simulink model "DisertatieVanca"  (R2022b)
settings: Solver=FixedStepAuto  StartTime=0.0  StopTime=10.0  RelTol=1e-3
values from neighbouring files (symbols this model uses):
  Ts = T_pwm    (= 0.001)    [RLagent.m]
  Ts_agent = Ts    (= 0.001)    [RLagent.m]
  Ts_speed = 10*Ts    (= 0.01)    [RLagent.m]
undefined symbols (not defined in the file or in its folder): DiscIntNeverNeededParam, Ion, Lithium
libraries: spsSeriesRLCBranchLib x10, spsDiodeLib x7, spsIGBTLib x6, mcbcontrolslib x3, simulink x3, spsVoltageMeasurementLib x3, spsThreePhaseVIMeasurementLib x3, spsCurrentMeasurementLib x2, spsBatteryLib x1, BatteryEstimators x1, spsIGBTDiodeLib x1, slpidlib x1
(part 1 of 2)
settings Model: Creator=uiv66426  LastModifiedBy=uiv66426
settings DebuggingCC: ParameterOverflowMsg=none  ParameterUnderflowMsg=error  ParameterPrecisionLossMsg=none
settings HardwareCC: TargetBitPerPointer=64  TargetBitPerSizeT=64  TargetBitPerPtrDiffT=64  TargetLongLongMode=on  TargetIntDivRoundTo=Zero  TargetEndianess=LittleEndian  TargetWordSize=64  TargetHWDeviceType=MATLAB Host  ProdEqTarget=off
settings RTWCC: Description=Rapid Simulation Target  SystemTargetFile=rsim.tlc  TemplateMakefile=rsim_default_tmf
settings RSimTargetCC: TargetLangStandard=C99 (ISO)  OptimizeReductions=off

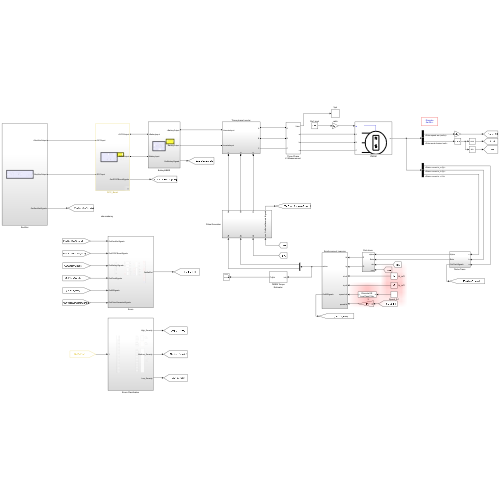
[thumbnail: Simulink's stored preview of the top-level diagram]
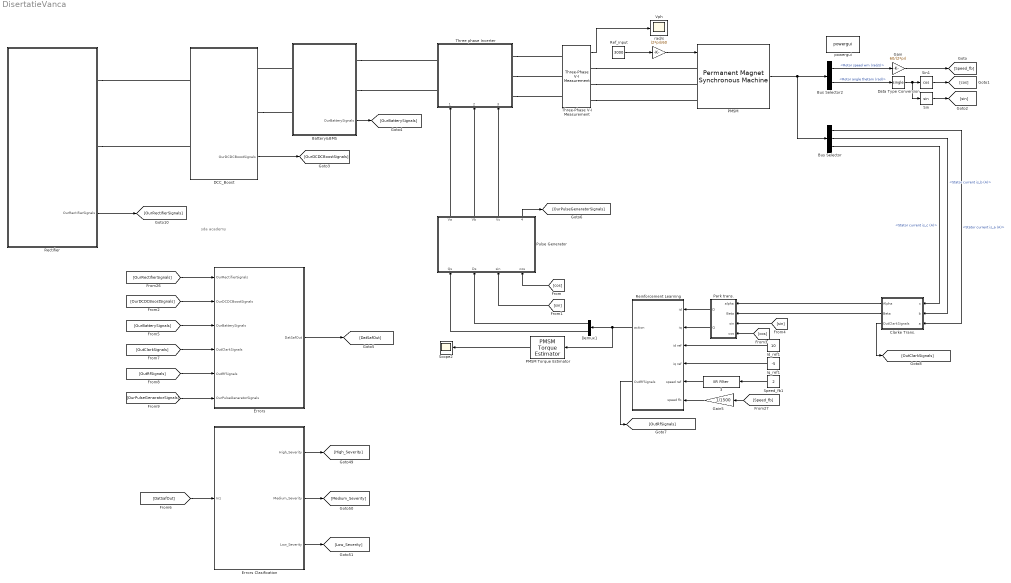
== system DisertatieVanca ==
  note: sda academy
  "   3" : mcbcontrolslib/IIR Filter  VariantControl=Low Pass Filter  VariantSelect=Low-pass  Filter_constant=0.01*(Ts_speed/Ts)  advancedSettings=off  Ts=50e-6  cutOff_freq=1
  Battery&BMS : Subsystem
      settings: PortSchema="{\"entries\":[{\"content\":{\"sides\":[{\"content\":{\"connectorIds\":[\"LConn1\",\"LConn2\"]},\"type\":\"ConnectorPlacement.EquallySpacedRectSide\",\"uuid\":\"cbc0bb53-0b94-40dd-8246-9b05db34f507\"},{\"content\":{\"connectorIds\":[\"RConn1\",\"RConn2\",\"Out1\"],\"side\":\"RIGHT\"},\"type\":\"ConnectorPlacement.EquallySpacedRectSide\",\"uuid\":\"2d021873-454e-497b-a321-1833202da2b2\"},{\"content\":{\"connectorIds\":[],\"side\":\"TOP\"},\"type\":\"ConnectorPlacement.EquallySpacedRectSide\",\"uuid\":\"d1b949f0-43da-4a40-bdda-1f67f09c131a\"}]},\"type\":\"ConnectorPlacement.EquallySpacedConnector\",\"uuid\":\"de95084d-4868-446f-8974-e187dacb7426\"}],\"packageUris\":[\"http://schema.mathworks.com/mf0/Connector/R2020b\"],\"version\":\"1.0\"}"
  Bus Selector : BusSelector  OutputSignals=Stator current is_a (A),Stator current is_b (A),Stator current is_c (A)
  Bus Selector2 : BusSelector  OutputSignals=Rotor speed wm (rad/s),Rotor angle thetam (rad)
  Clarke Trans. : Subsystem
  DCC_Boost : Subsystem
      settings: PortSchema="{\"entries\":[{\"content\":{\"sides\":[{\"content\":{\"connectorIds\":[\"LConn1\",\"LConn2\"]},\"type\":\"ConnectorPlacement.EquallySpacedRectSide\",\"uuid\":\"cbc0bb53-0b94-40dd-8246-9b05db34f507\"},{\"content\":{\"connectorIds\":[\"RConn1\",\"RConn2\",\"Out1\"],\"side\":\"RIGHT\"},\"type\":\"ConnectorPlacement.EquallySpacedRectSide\",\"uuid\":\"2d021873-454e-497b-a321-1833202da2b2\"},{\"content\":{\"connectorIds\":[],\"side\":\"TOP\"},\"type\":\"ConnectorPlacement.EquallySpacedRectSide\",\"uuid\":\"d1b949f0-43da-4a40-bdda-1f67f09c131a\"}]},\"type\":\"ConnectorPlacement.EquallySpacedConnector\",\"uuid\":\"de95084d-4868-446f-8974-e187dacb7426\"}],\"packageUris\":[\"http://schema.mathworks.com/mf0/Connector/R2020b\"],\"version\":\"1.0\"}"
  Data Type Conversion : DataTypeConversion  OutDataTypeStr=single  SaturateOnIntegerOverflow=off  RndMeth=Floor
  Demux1 : Demux  Outputs=2
  Errors : Subsystem
  Errors Clasification : Subsystem
  Gain : Gain  Gain=60/(2*pi)  OutDataTypeStr=double
  Gain5 : Gain  Gain=1/1500
  Id_ref1 : Constant  Value=10  OutDataTypeStr=double  SampleTime=Ts_speed
  Iq_ref1 : Constant  Value=-5  OutDataTypeStr=double  SampleTime=Ts_speed
  PMSM : spsPermanentMagnetSynchronousMachineLib/Permanent Magnet Synchronous Machine  NbPhases=3  FluxDistribution=Sinusoidal  RotorType=Salient-pole  MechanicalLoad=Speed w  PresetModel=No  ShowDetailedParameters=on  MeasurementBus=off  Resistance=18.7  Inductance=8.5e-3  dqInductances=[0.02547 0.02816]  La=0.000395  MachineConstant=Flux linkage established by magnets (V.s)  Flux=0.1716  VoltageCst=62.2496  TorqueCst=0.5148  Flat=120  Mechanical=[2.26e-05 1.349e-05 2 0]  PolePairs=2  InitialConditions=[0,0, 0,0]  InitialConditions5ph=[0 0 0 0 0 0]  RefAngle=Aligned with phase A axis (original Park)  IterativeDiscreteModel=Trapezoidal non iterative  TsBlock=-1  TsPowergui=0
  PMSM Torque Estimator : eePmsmTorqueEstimator/PMSM Torque Estimator  ParamType=Constant parameters  p=8  idVect=[-200, 200]  iqVect=[-200, 200]  LdMatrix=0.0002 * ones(2, 2)  LqMatrix=0.0002 * ones(2, 2)  psimMatrix=0.04 * ones(2, 2)  Ld=0.0002  Lq=0.0002  psim=0.04  Ts=-1
  Park trans. : Subsystem
  Pulse Generator : Subsystem
  Rectifier : Subsystem
      settings: PortSchema="{\"entries\":[{\"content\":{\"sides\":[{\"content\":{\"connectorIds\":[]},\"type\":\"ConnectorPlacement.EquallySpacedRectSide\",\"uuid\":\"7d3ba707-0ee8-4d26-a752-be0b8f38d830\"},{\"content\":{\"connectorIds\":[\"RConn1\",\"RConn2\",\"Out1\"],\"side\":\"RIGHT\"},\"type\":\"ConnectorPlacement.EquallySpacedRectSide\",\"uuid\":\"4da73b4e-8794-485b-9d0a-8f3b9b630819\"},{\"content\":{\"connectorIds\":[],\"side\":\"TOP\"},\"type\":\"ConnectorPlacement.EquallySpacedRectSide\",\"uuid\":\"189264b5-1a07-455a-ade0-b52dce53e5ab\"}]},\"type\":\"ConnectorPlacement.EquallySpacedConnector\",\"uuid\":\"df5a9191-3afb-48d4-8cb4-bd3682c9bea9\"}],\"packageUris\":[\"http://schema.mathworks.com/mf0/Connector/R2020b\"],\"version\":\"1.0\"}"
  Ref_input : Constant  Value=3000  SampleTime=0.0005
  Reinforcement Learning : Subsystem
  Scope2 : Scope
  Sin : Trigonometry  NumberOfDataPoints=double
  Sin1 : Trigonometry  Operator=cos
  Speed_fb1 : Constant  Value=2  SampleTime=Ts_speed
  Three phase Inverter : Subsystem
      settings: PortSchema="{\"entries\":[{\"content\":{\"sides\":[{\"content\":{\"connectorIds\":[\"LConn1\",\"LConn2\"]},\"type\":\"ConnectorPlacement.EquallySpacedRectSide\",\"uuid\":\"7b196236-775e-42c1-83d0-0d6d250710e6\"},{\"content\":{\"connectorIds\":[\"RConn1\",\"RConn2\",\"RConn3\"],\"side\":\"RIGHT\"},\"type\":\"ConnectorPlacement.EquallySpacedRectSide\",\"uuid\":\"b457e177-0c4c-43e7-9cb7-fdd2074136b6\"},{\"content\":{\"connectorIds\":[],\"side\":\"TOP\"},\"type\":\"ConnectorPlacement.EquallySpacedRectSide\",\"uuid\":\"18a8f709-510a-4ef1-9b8b-174ec6aa79c3\"},{\"content\":{\"connectorIds\":[\"In1\",\"In2\",\"In3\"],\"side\":\"BOTTOM\"},\"type\":\"ConnectorPlacement.EquallySpacedRectSide\",\"uuid\":\"6b6fe34a-9a26-41fc-be3f-ad32a70b0e9c\"}]},\"type\":\"ConnectorPlacement.EquallySpacedConnector\",\"uuid\":\"c4aeab25-f1ae-4405-83d3-42d09976eee9\"}],\"packageUris\":[\"http://schema.mathworks.com/mf0/Connector/R2020b\"],\"version\":\"1.0\"}"
  "Three-Phase V-I Measurement " : spsThreePhaseVIMeasurementLib/Three-Phase V-I Measurement  VoltageMeasurement=phase-to-phase  SetLabelV=off  LabelV=Vabc  Vpu=off  VpuLL=off  CurrentMeasurement=no  SetLabelI=off  LabelI=Iabc  Ipu=off  Pbase=100e6  Vbase=500e3  OutputType=Complex  PhasorSimulation=off  PSBequivalent=0
  Vph : Scope
  powergui : spspowerguiLib/powergui  Priority=1  SimulationMode=Discrete  SampleTime=50e-6  frequency=60  Iterations=50  frequencyindice=0  Pbase=100e6  ErrMax=1e-4  UnitsV=kV  UnitsW=MW  buscounter=0  FunctionMessages=off  echomessages=off  EnableUseOfTLC=off  CurrentSourceSwitches=off  DisableSnubberDevices=off  DisableRonSwitches=off  DisableVfSwitches=off  DisplayEquations=off  AutomaticDiscreteSolvers=off  SolverType=Tustin/Backward Euler (TBE)  Interpol=off  ExternalGateDelay=off  methode=off  Ts=100  x0status=blocks  SPID=on  SwTol=0  HookPort=off  NonlinearTolerance=1e-4  nMaxIteration=100  ContinueOnMaxIteration=off  RestoreLinks=warning  ResistiveCurrentMeasurement=off  Frange=[0:2:500]  Ylog=off  Xlog=on  ShowGrid=off  save=off  variable=ZData  structure=0  ZoomFFT=off  StartTime=0.0  cycles=1  DisplayStyle=1  fundamental=60  FreqAxis=off  MaxFrequency=1000  frequencyindicesteady=1  RmsSteady=1  display=off
  rad/s : Gain  Gain=(2*pi)/60  OutDataTypeStr=double
  wires:
  Ref_input/1 -> rad/s/1
  rad/s/1 -> PMSM/1
  [cos] -> Park trans./4(cos)
  Sin1/1 -> [cos]
  [sin] -> Park trans./3(sin)
  Bus Selector/3 -> Clarke Trans./1(c)  "<Stator current is_c (A)>"
  Clarke Trans./2(Beta) -> Park trans./2(Beta)
  Bus Selector/1 -> Clarke Trans./3(a)  "<Stator current is_a (A)>"
  Sin/1 -> [sin]
  Bus Selector/2 -> Clarke Trans./2(b)  "<Stator current is_b (A)>"
  Gain/1 -> [Speed_fb]
  Data Type Conversion/1 -> Sin/1, Sin1/1
  Clarke Trans./1(Alpha) -> Park trans./1(alpha)
  Bus Selector2/1 -> Gain/1  "<Rotor speed wm (rad/s)>"
  PMSM/1 -> Bus Selector/1, Bus Selector2/1
  "Three-Phase V-I Measurement "/1 -> Vph/1
  [cos] -> Pulse Generator/4(cos)
  [sin] -> Pulse Generator/3(sin)
  Park trans./1(D) -> Reinforcement Learning/1(id)
  Park trans./2(Q) -> Reinforcement Learning/2(iq)
  Gain5/1 -> Reinforcement Learning/6(speed fb)
  [Speed_fb] -> Gain5/1
  Iq_ref1/1 -> Reinforcement Learning/4(iq ref)
  "   3"/1 -> Reinforcement Learning/5(speed ref)
  Speed_fb1/1 -> "   3"/1
  Id_ref1/1 -> Reinforcement Learning/3(id ref)
  PMSM Torque Estimator/1 -> Scope2/1
  Reinforcement Learning/1(action) -> PMSM Torque Estimator/1, Demux1/1
  Demux1/1 -> Pulse Generator/2(Ds)
  Demux1/2 -> Pulse Generator/1(Qs)
  Rectifier/1(OurRectifierSignals) -> [OurRectifierSignals]
  DCC_Boost/1(OurDCDCBoostSignals) -> [OurDCDCBoostSignals]
  Battery&BMS/1(OurBatterySignals) -> [OurBatterySignals]
  [OurRectifierSignals] -> Errors/1(OurRectifierSignals)
  [OurDCDCBoostSignals] -> Errors/2(OurDCDCBoostSignals)
  [OurBatterySignals] -> Errors/3(OurBatterySignals)
  Pulse Generator/4(OurPulseGenaratorSignals) -> [OurPulseGenaratorSignals]
  Reinforcement Learning/2(OutRfSignals) -> [OutRfSignals]
  Clarke Trans./3(OutClarkSignals) -> [OutClarkSignals]
  [OutClarkSignals] -> Errors/4(OutClarkSignals)
  [OutRfSignals] -> Errors/5(OutRfSignals)
  [OurPulseGenaratorSignals] -> Errors/6(OurPulseGenaratorSignals)
  Errors/1(DatSafOut) -> [DatSafOut]
  [DatSafOut] -> Errors Clasification/1(In1)
  Errors Clasification/3(Low_Severity) -> [Low_Severity]
  Errors Clasification/2(Medium_Severity) -> [Medium_Severity]
  Errors Clasification/1(High_Severity) -> [High_Severity]
  Pulse Generator/1(Va) -> Three phase Inverter/1(1)
  Pulse Generator/2(Vb) -> Three phase Inverter/2(2)
  Pulse Generator/3(Vc) -> Three phase Inverter/3(3)
  Bus Selector2/2 -> Data Type Conversion/1  "<Rotor angle thetam (rad)>"
  connections:
  Three phase Inverter/RConn3 -- "Three-Phase V-I Measurement "/LConn3
  Three phase Inverter/RConn1 -- "Three-Phase V-I Measurement "/LConn1
  Three phase Inverter/RConn2 -- "Three-Phase V-I Measurement "/LConn2
  "Three-Phase V-I Measurement "/RConn2 -- PMSM/LConn2
  "Three-Phase V-I Measurement "/RConn3 -- PMSM/LConn3
  Rectifier/RConn1 -- DCC_Boost/LConn1
  Rectifier/RConn2 -- DCC_Boost/LConn2
  Battery&BMS/LConn1 -- DCC_Boost/RConn1
  DCC_Boost/RConn2 -- Battery&BMS/LConn2
  Battery&BMS/RConn1 -- Three phase Inverter/LConn1
  Battery&BMS/RConn2 -- Three phase Inverter/LConn2
  "Three-Phase V-I Measurement "/RConn1 -- PMSM/LConn1

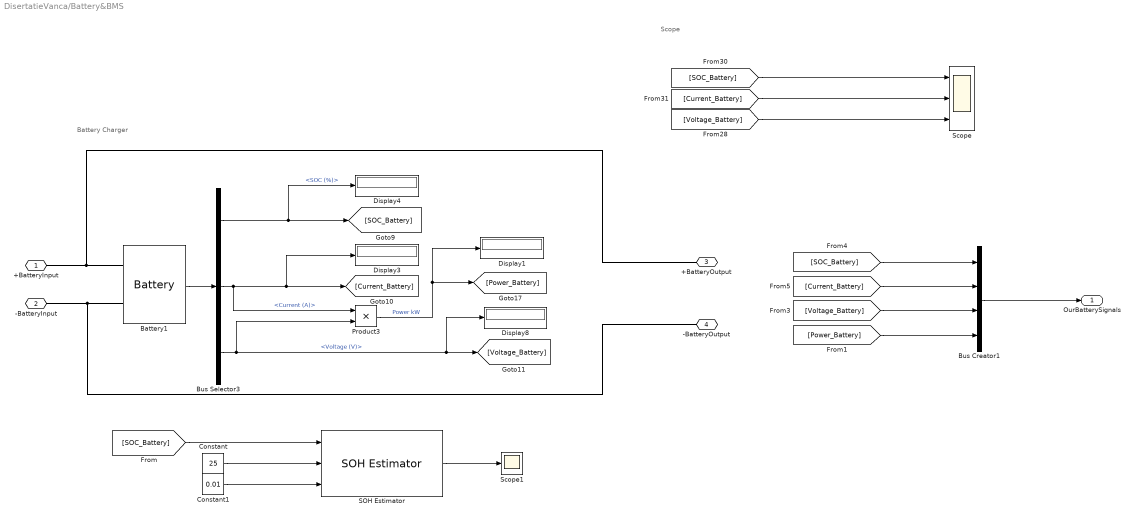
== system DisertatieVanca/Battery&BMS ==
  note: Battery Charger
  note: Scope
  Battery1 : spsBatteryLib/Battery  BatType=Lithium-Ion  ShowTempParam=off  ThermalPreset=no  ShowAgeParam=off  NomV=800  NomQ=116.75  SOC=100  Batt_Tr=10  PresetModel=on  MaxQ=116.75  MinV=600  FullV=931.1897  Dis_rate=50.7609  R=0.068522  Normal_OP=105.5826  expZone="[864.3087      5.735978]"  current=[17]  Units=Time  Tci=20  NomT=20  T2=-30  MaxQ2=4.8  FullV2=7.1  Normal_OP2=5.655  expZone2="[6.58           1]"  Rca=0.6  ti=2000  Dp=0  Neq0=0  Tsim=1e6  Ta1=25  Qeol=5.4*0.9  Reol=0.013333*1.2  Char_age=[2.3478, 3]  Dis_age=[2.3478, 10]  N1=1500  N2=10500  N3=1000  N4=1400  Ta2=45  N5=950
      settings: LibrarySourceBlock=electricdrivelib/Extra Sources/Battery
  Bus Creator1 : BusCreator  Inputs=4
  Bus Selector3 : BusSelector  OutputSignals=SOC (%),Current (A),Voltage (V)
  Constant : Constant  Value=25  SampleTime=-1
  Constant1 : Constant  Value=0.01  SampleTime=-1
  Display{1,3..4,8} (4 alike) : Display
  Product3 : Product
  SOH Estimator : BatteryEstimators/SOH Estimator  SOC_vec=[0, .1, .25, .5, .75, .9, 1]  T_vec=[278, 293, 313]  R0_new_mat=[.0117, .0085, .009; .011, .0085, .009; .0114, .0087, .0092; .0107, .0082, .0088; .0107, .0083, .0091; .0113, .0085, .0089; .0116, .0085, .0089]  R0_EOL_mat=[.0234,.017,.018;.022,.017,.018;.0228,.0174,.0184;.0214,.0164,.0176;.0214,.0166,.0182;.0226,.017,.0178;.0232,.017,.0178]
      settings: LibrarySourceBlock=batt_sl_lib/Estimators/SOH Estimator
  Scope : Scope  NumInputPorts=3
  Scope1 : Scope
  +BatteryInput : PMIOPort  Side=Left
  -BatteryInput : PMIOPort  Port=2  Side=Left
  +BatteryOutput : PMIOPort  Port=3  Side=Right
  -BatteryOutput : PMIOPort  Port=4  Side=Right
  OurBatterySignals : Outport
  wires:
  Bus Selector3/1 -> Display4/1, [SOC_Battery]  "<SOC (%)>"
  Product3/1 -> Display1/1, [Power_Battery]  "Power kW"
  Bus Selector3/2 -> Product3/1, Display3/1, [Current_Battery]  "<Current (A)>"
  Battery1/1 -> Bus Selector3/1
  Bus Selector3/3 -> Product3/2, Display8/1, [Voltage_Battery]  "<Voltage (V)>"
  [SOC_Battery] -> Scope/1
  [Current_Battery] -> Scope/2
  [Voltage_Battery] -> Scope/3
  [SOC_Battery] -> Bus Creator1/1
  [Power_Battery] -> Bus Creator1/4
  Bus Creator1/1 -> OurBatterySignals/1
  [Current_Battery] -> Bus Creator1/2
  [Voltage_Battery] -> Bus Creator1/3
  Constant/1 -> SOH Estimator/2
  Constant1/1 -> SOH Estimator/3
  [SOC_Battery] -> SOH Estimator/1
  SOH Estimator/1 -> Scope1/1
  connections:
  Battery1/LConn2 -- -BatteryOutput/RConn1 -- -BatteryInput/RConn1
  Battery1/LConn1 -- +BatteryOutput/RConn1 -- +BatteryInput/RConn1

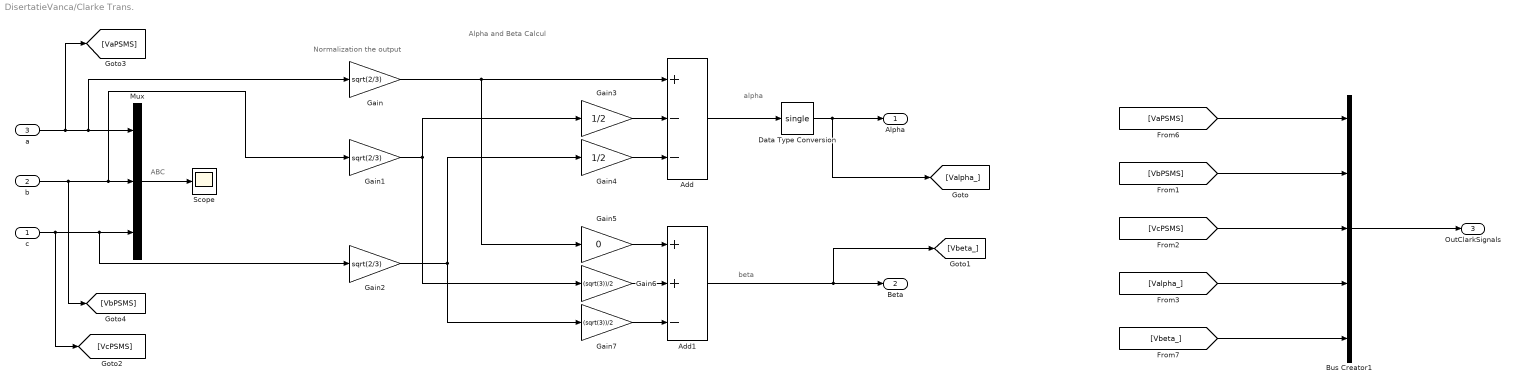
== system DisertatieVanca/Clarke Trans. ==
  note: ABC
  note: beta
  note: alpha
  note: Normalization the output
  note: Alpha and Beta Calcul
  c : Inport
  b : Inport  Port=2
  a : Inport  Port=3
  Add : Sum  Inputs=+--  AccumDataTypeStr=single
  Add1 : Sum  Inputs=++-  AccumDataTypeStr=double
  Bus Creator1 : BusCreator  Inputs=5
  Data Type Conversion : DataTypeConversion  OutDataTypeStr=single  SaturateOnIntegerOverflow=off  RndMeth=Floor
  Gain : Gain  Gain=sqrt(2/3)
  Gain1 : Gain  Gain=sqrt(2/3)
  Gain2 : Gain  Gain=sqrt(2/3)
  Gain3 : Gain  Gain=1/2
  Gain4 : Gain  Gain=1/2
  Gain5 : Gain  Gain=0
  Gain6 : Gain  Gain=(sqrt(3))/2
  Gain7 : Gain  Gain=(sqrt(3))/2
  Mux : Mux  Inputs=3
  Scope : Scope
  Alpha : Outport
  Beta : Outport  Port=2
  OutClarkSignals : Outport  Port=3
  wires:
  Gain2/1 -> Gain7/1, Gain4/1
  Gain/1 -> Gain5/1, Add/1
  Gain1/1 -> Gain6/1, Gain3/1
  Gain6/1 -> Add1/2
  a/1 -> [VaPSMS], Gain/1, Mux/1
  b/1 -> [VbPSMS], Gain1/1, Mux/2
  c/1 -> [VcPSMS], Gain2/1, Mux/3
  Gain5/1 -> Add1/1
  Gain7/1 -> Add1/3
  Gain3/1 -> Add/2
  Gain4/1 -> Add/3
  Mux/1 -> Scope/1
  Add1/1 -> [Vbeta_], Beta/1
  Add/1 -> Data Type Conversion/1
  Data Type Conversion/1 -> [Valpha_], Alpha/1
  [VaPSMS] -> Bus Creator1/1
  [Vbeta_] -> Bus Creator1/5
  Bus Creator1/1 -> OutClarkSignals/1
  [VcPSMS] -> Bus Creator1/3
  [VbPSMS] -> Bus Creator1/2
  [Valpha_] -> Bus Creator1/4

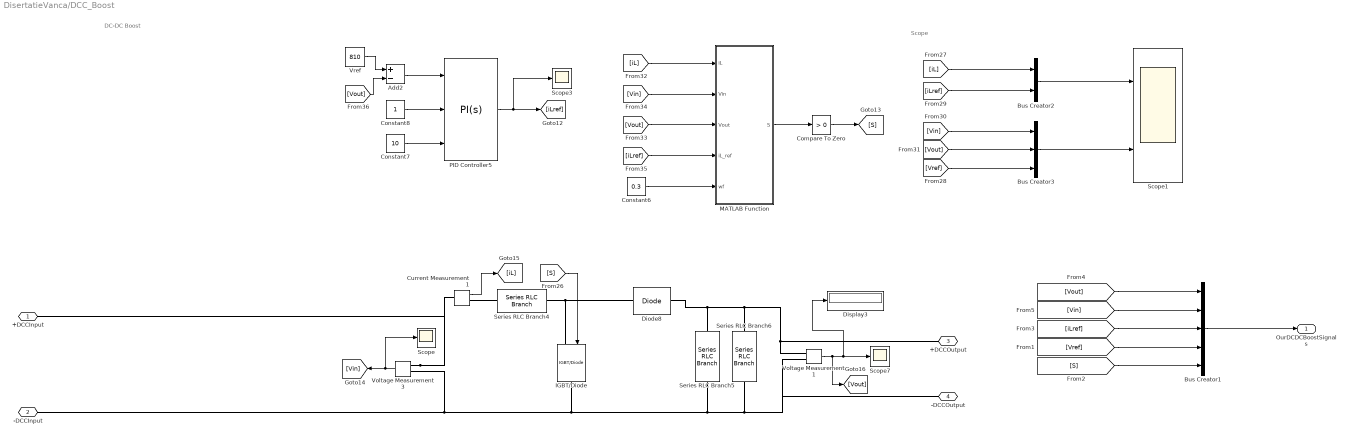
== system DisertatieVanca/DCC_Boost ==
  note: DC-DC Boost
  note: Scope
  Add2 : Sum  Inputs=+-
  Bus Creator1 : BusCreator  Inputs=5
  Bus Creator2 : BusCreator  Inputs=2
  Bus Creator3 : BusCreator  Inputs=3
  Compare To Zero : simulink/Logic and Bit Operations/Compare To Zero  relop=>  OutDataTypeStr=boolean
  Constant6 : Constant  Value=0.3
  Constant7 : Constant  Value=10
  Constant8 : Constant
  Current Measurement1 : spsCurrentMeasurementLib/Current Measurement  PhasorSimulation=off  OutputType=Complex  PSBequivalent=0
  Diode8 : spsDiodeLib/Diode  Ron=0.005  Lon=0  Vf=0.8  IC=0  UseSnubber=0  Rs=500  Cs=250e-9  Measurements=off
  Display3 : Display
  IGBT/Diode : spsIGBTDiodeLib/IGBT//Diode  Ron=1e-3  Rs=1e5  Cs=inf  Measurements=off
  MATLAB Function : MATLAB Function  TreatAsAtomicUnit=on
  PID Controller5 : slpidlib/PID Controller  Controller=PI  Form=Parallel  TimeDomain=Continuous-time  UseExternalTs=off  SampleTime=-1  IntegratorMethod=Forward Euler  FilterMethod=Forward Euler  ControllerParametersSource=external  P=1  I=1  UseKiTs=off  D=0  N=100  UseFilter=on  TunerSelectOption=Transfer Function Based (PID Tuner App)  InitialConditionSource=internal  InitialConditionForIntegrator=0  InitialConditionForFilter=0  DifferentiatorICPrevScaledInput=0  ExternalReset=none  TrackingMode=off  Kt=1  LimitOutput=off  SatLimitsSource=internal  UpperSaturationLimit=inf  LowerSaturationLimit=-inf  LinearizeAsGain=on  AntiWindupMode=none  Kb=1  LimitIntegrator=off  UpperIntegratorSaturationLimit=inf  LowerIntegratorSaturationLimit=-inf  POutMin=[]  POutMax=[]  IOutMin=[]  IOutMax=[]  DOutMin=[]  DOutMax=[]  NOutMin=[]  NOutMax=[]  SumOutMin=[]  SumOutMax=[]  SaturationOutMin=[]  SaturationOutMax=[]  PParamMin=[]  PParamMax=[]  IParamMin=[]  IParamMax=[]  DParamMin=[]  DParamMax=[]  NParamMin=[]  NParamMax=[]  KbParamMin=[]  KbParamMax=[]  KtParamMin=[]  KtParamMax=[]  KbOutMin=[]  KbOutMax=[]  KtOutMin=[]  KtOutMax=[]  IntegratorOutMin=[]  IntegratorOutMax=[]  FilterOutMin=[]  FilterOutMax=[]  SumI1OutMin=[]  SumI1OutMax=[]  SumI2OutMin=[]  SumI2OutMax=[]  SumI3OutMin=[]  SumI3OutMax=[]  SumI4OutMin=[]  SumI4OutMax=[]  SumDOutMin=[]  SumDOutMax=[]  DifferentiatorOutMin=[]  DifferentiatorOutMax=[]  FilterDiffOutCoefMin=[]  FilterDiffOutCoefMax=[]  ReciprocalOutMin=[]  ReciprocalOutMax=[]  SumDenOutMin=[]  SumDenOutMax=[]  SumNumOutMin=[]  SumNumOutMax=[]  DivideOutMin=[]  DivideOutMax=[]  UdiffTsProdOutMin=[]  UdiffTsProdOutMax=[]  NTsProdOutMin=[]  NTsProdOutMax=[]  UintegralTsProdOutMin=[]  UintegralTsProdOutMax=[]  UngainTsProdOutMin=[]  UngainTsProdOutMax=[]  ClampingZeroOutDataTypeStr=Inherit: Inherit via back propagation  ClampingZeroOutMin=[]  ClampingZeroOutMax=[]  FilterDenConstantOutDataTypeStr=Inherit: Inherit via back propagation  FilterDenConstantOutMin=[]  FilterDenConstantOutMax=[]  PCopyOutDataTypeStr=Inherit: Inherit via back propagation  PCopyOutMin=[]  PCopyOutMax=[]  NCopyOutDataTypeStr=Inherit: Inherit via back propagation  NCopyOutMin=[]  NCopyOutMax=[]  IntegratorContinuousStateAttributes=''  IntegratorStateMustResolveToSignalObject=off  IntegratorRTWStateStorageClass=Auto  FilterContinuousStateAttributes=''  FilterStateMustResolveToSignalObject=off  FilterRTWStateStorageClass=Auto  ParallelPVariant=ExternalParameters  IdealPVariant=Disabled  IVariant=ExternalParameters  DVariant=Disabled  IntegratorVariant=Continuous  SatVariant=Disabled  AWVariant=Passthrough  PCopyVariant=Disabled  TRVariant=Disabled  FdbkBlocksVariant=Forward  IdealPFdbkVariant=Disabled  SatFdbkVariant=Disabled  DerivativeFilterVariant=Disabled  NVariant=Disabled  NCopyVariant=Disabled_SignalSpec  FilterICVariant=Disabled  IntegratorICVariant=InternalICs  ExternalResetVariant=Disabled  TRSumVariant=Passthrough  SumFdbkVariant=Disabled  SumVariant=Sum_PI  TsampFilterVariant=InternalTs  TsampNgainVariant=Passthrough  TsampIntegralVariant=Passthrough  ExternalSaturationOutDataTypeStr=Inherit: Same as second input
  Scope : Scope
  Scope1 : Scope  NumInputPorts=2
  Scope3 : Scope
  Scope7 : Scope
  Series RLC Branch4 : spsSeriesRLCBranchLib/Series RLC Branch  LConnTagsString=__new0  RConnTagsString=__new0  BranchType=RL  Resistance=1.5  Inductance=0.003  SetiL0=off  InitialCurrent=0  Capacitance=200e-6  Setx0=off  InitialVoltage=0  Measurements=None
  Series RLC Branch5 : spsSeriesRLCBranchLib/Series RLC Branch  LConnTagsString=__new0  RConnTagsString=__new0  BranchType=C  Resistance=1  Inductance=0.003  SetiL0=off  InitialCurrent=0  Capacitance=0.005  Setx0=off  InitialVoltage=0  Measurements=None
  Series RLC Branch6 : spsSeriesRLCBranchLib/Series RLC Branch  LConnTagsString=__new0  RConnTagsString=__new0  BranchType=R  Resistance=1.17  Inductance=0.003  SetiL0=off  InitialCurrent=0  Capacitance=0.006  Setx0=off  InitialVoltage=0  Measurements=None
  Voltage Measurement1 : spsVoltageMeasurementLib/Voltage Measurement  PhasorSimulation=off  OutputType=Complex  PSBequivalent=0
  Voltage Measurement3 : spsVoltageMeasurementLib/Voltage Measurement  PhasorSimulation=off  OutputType=Complex  PSBequivalent=0
  Vref : Constant  Value=810
  +DCCInput : PMIOPort  Side=Left
  -DCCInput : PMIOPort  Port=2  Side=Left
  +DCCOutput : PMIOPort  Port=3  Side=Right
  -DCCOutput : PMIOPort  Port=4  Side=Right
  OurDCDCBoostSignals : Outport
  wires:
  [iLref] -> MATLAB Function/4(iL_ref)
  MATLAB Function/1(S) -> Compare To Zero/1
  [Vout] -> Add2/2
  Current Measurement1/1 -> [iL]
  [iL] -> Bus Creator2/1
  [S] -> IGBT/Diode/1
  [Vout] -> Bus Creator3/2
  PID Controller5/1 -> Scope3/1, [iLref]
  Constant8/1 -> PID Controller5/2
  [iL] -> MATLAB Function/1(iL)
  Bus Creator2/1 -> Scope1/1
  Bus Creator3/1 -> Scope1/2
  Constant7/1 -> PID Controller5/3
  [iLref] -> Bus Creator2/2
  [Vin] -> Bus Creator3/1
  Voltage Measurement1/1 -> [Vout], Display3/1, Scope7/1
  Add2/1 -> PID Controller5/1
  [Vref] -> Bus Creator3/3
  Voltage Measurement3/1 -> Scope/1, [Vin]
  Vref/1 -> Add2/1
  [Vout] -> MATLAB Function/3(Vout)
  Compare To Zero/1 -> [S]
  Constant6/1 -> MATLAB Function/5(wf)
  [Vin] -> MATLAB Function/2(Vin)
  [S] -> Bus Creator1/5
  [Vin] -> Bus Creator1/2
  Bus Creator1/1 -> OurDCDCBoostSignals/1
  [Vout] -> Bus Creator1/1
  [iLref] -> Bus Creator1/3
  [Vref] -> Bus Creator1/4
  connections:
  Voltage Measurement1/LConn1 -- +DCCOutput/RConn1 -- Series RLC Branch6/LConn1 -- Diode8/RConn1 -- Series RLC Branch5/LConn1
  Series RLC Branch4/RConn1 -- IGBT/Diode/LConn1 -- Diode8/LConn1
  Voltage Measurement3/LConn2 -- IGBT/Diode/RConn1 -- -DCCOutput/RConn1 -- Voltage Measurement1/LConn2 -- Series RLC Branch6/RConn1 -- Series RLC Branch5/RConn1 -- -DCCInput/RConn1
  Current Measurement1/RConn1 -- Series RLC Branch4/LConn1
  Voltage Measurement3/LConn1 -- Current Measurement1/LConn1 -- +DCCInput/RConn1

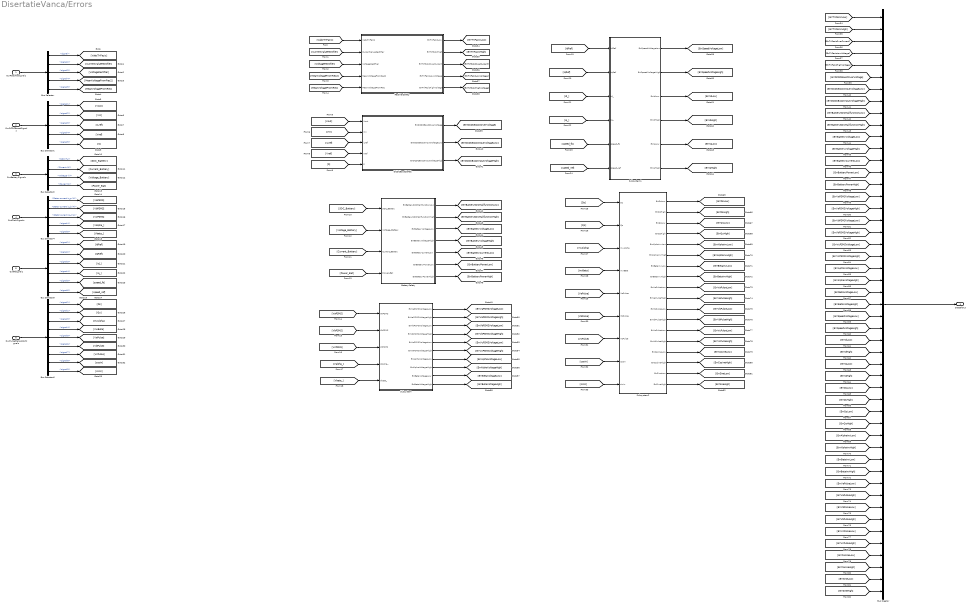
== system DisertatieVanca/Errors ==
  OurRectifierSignals : Inport
  OurDCDCBoostSignals : Inport  Port=2
  OurBatterySignals : Inport  Port=3
  OutClarkSignals : Inport  Port=4
  OutRfSignals : Inport  Port=5
  OurPulseGenaratorSignals : Inport  Port=6
  BatterySafety : Subsystem
  Bus Creator : BusCreator  Inputs=49
  Bus Selector : BusSelector  OutputSignals=signal,signal2,signal3,signal4,signal5
  Bus Selector1 : BusSelector  OutputSignals=signal1,signal2,signal3,signal4,signal5
  Bus Selector2 : BusSelector  OutputSignals=SOC (%),Current (A),Voltage (V),Power kW
  Bus Selector4 : BusSelector  OutputSignals=Stator current is_a (A),Stator current is_b (A),Stator current is_c (A),signal4,signal5
  Bus Selector5 : BusSelector  OutputSignals=signal1,signal2,signal3,signal4,signal5,signal6
  Bus Selector6 : BusSelector  OutputSignals=signal1,signal2,signal3,signal4,signal5,signal6,signal7,signal8,signal9
  DCDCBoostSafety : Subsystem
  RectifierSafety : Subsystem
  Subsystem : Subsystem
  Subsystem1 : Subsystem
  Subsystem2 : Subsystem
  DatSafOut : Outport
  wires:
  OurRectifierSignals/1 -> Bus Selector/1
  OurDCDCBoostSignals/1 -> Bus Selector1/1
  OurBatterySignals/1 -> Bus Selector2/1
  OutClarkSignals/1 -> Bus Selector4/1
  OutRfSignals/1 -> Bus Selector5/1
  OurPulseGenaratorSignals/1 -> Bus Selector6/1
  Bus Selector/1 -> [VabcTriFazic]  "<signal>"
  Bus Selector/2 -> [CurrentValueRectifier]  "<signal2>"
  Bus Selector/3 -> [VoltageRectifier]  "<signal3>"
  Bus Selector/4 -> [MeanVoltageFromRec2]  "<signal4>"
  Bus Selector/5 -> [MeanVoltageFromRec]  "<signal5>"
  Bus Selector1/1 -> [Vout]  "<signal1>"
  Bus Selector1/2 -> [Vin]  "<signal2>"
  Bus Selector1/3 -> [iLref]  "<signal3>"
  Bus Selector1/4 -> [Vref]  "<signal4>"
  Bus Selector1/5 -> [S]  "<signal5>"
  Bus Selector2/1 -> [SOC_Battery]  "<SOC (%)>"
  Bus Selector2/2 -> [Current_Battery]  "<Current (A)>"
  Bus Selector2/3 -> [Voltage_Battery]  "<Voltage (V)>"
  Bus Selector2/4 -> [Power_Bat]  "<Power kW>"
  Bus Selector4/1 -> [VaPSMS]  "<Stator current is_a (A)>"
  Bus Selector4/2 -> [VbPSMS]  "<Stator current is_b (A)>"
  Bus Selector4/3 -> [VcPSMS]  "<Stator current is_c (A)>"
  Bus Selector4/4 -> [Valpha_]  "<signal4>"
  Bus Selector4/5 -> [Vbeta_]  "<signal5>"
  Bus Selector5/1 -> [IdRef]  "<signal1>"
  Bus Selector5/2 -> [IqRef]  "<signal2>"
  Bus Selector5/3 -> [Id_]  "<signal3>"
  Bus Selector5/4 -> [Iq_]  "<signal4>"
  Bus Selector5/5 -> [speed_fb]  "<signal5>"
  Bus Selector5/6 -> [speed_ref]  "<signal6>"
  Bus Selector6/1 -> [Ds]  "<signal1>"
  Bus Selector6/2 -> [Qs]  "<signal2>"
  Bus Selector6/3 -> [InvAlpha]  "<signal3>"
  Bus Selector6/4 -> [InvBeta]  "<signal4>"
  Bus Selector6/5 -> [VaPulse]  "<signal5>"
  Bus Selector6/6 -> [VbPulse]  "<signal6>"
  Bus Selector6/7 -> [VcPulse]  "<signal7>"
  Bus Selector6/8 -> [cosIn]  "<signal8>"
  Bus Selector6/9 -> [sinIn]  "<signal9>"
  [VabcTriFazic] -> RectifierSafety/1(VabcTriFazic)
  [CurrentValueRectifier] -> RectifierSafety/2(CurrentValueRectifier)
  [VoltageRectifier] -> RectifierSafety/3(VoltageRectifier)
  [MeanVoltageFromRec2] -> RectifierSafety/4(MeanVoltageFromRec2)
  [MeanVoltageFromRec] -> RectifierSafety/5(MeanVoltageFromRec)
  RectifierSafety/1(ErrTriFazicLow) -> [ErrTriFazicLow]
  RectifierSafety/3(ErrTriFazicOverCurrent) -> [ErrTriFazicOverCurrent]
  RectifierSafety/4(ErrTriFazicLowVoltage) -> [ErrTriFazicLowVoltage]
  RectifierSafety/5(ErrTriFazicHighVoltage) -> [ErrTriFazicHighVoltage]
  Bus Creator/1 -> DatSafOut/1
  [Vout] -> DCDCBoostSafety/1(Vout)
  [Vin] -> DCDCBoostSafety/2(Vin)
  [iLref] -> DCDCBoostSafety/3(iLref)
  [Vref] -> DCDCBoostSafety/4(Vref)
  [S] -> DCDCBoostSafety/5(S)
  DCDCBoostSafety/1(ErrDCDCBoostOverVoltage) -> [ErrDCDCBoostOverVoltage]
  DCDCBoostSafety/2(ErrDCDCBoostInputVoltageLow) -> [ErrDCDCBoostInputVoltageLow]
  DCDCBoostSafety/3(ErrDCDCBoostInputVoltageHigh) -> [ErrDCDCBoostInputVoltageHigh]
  [SOC_Battery] -> BatterySafety/1(SOC_Battery)
  [Current_Battery] -> BatterySafety/3(Current_Battery)
  [Voltage_Battery] -> BatterySafety/2(Voltage_Battery)
  [Power_Bat] -> BatterySafety/4(Power_Bat)
  [VaPSMS] -> Subsystem/1(VaPSMS)
  [VbPSMS] -> Subsystem/2(VbPSMS)
  [Vbeta_] -> Subsystem/5(Vbeta_)
  [Valpha_] -> Subsystem/4(Valpha_)
  [VcPSMS] -> Subsystem/3(VcPSMS)
  [IdRef] -> Subsystem1/1(IdRef)
  [IqRef] -> Subsystem1/2(IqRef)
  [Id_] -> Subsystem1/3(Id_)
  [Iq_] -> Subsystem1/4(Iq_)
  [speed_fb] -> Subsystem1/5(speed_fb)
  [speed_ref] -> Subsystem1/6(speed_ref)
  BatterySafety/1(ErrBatterySOCMallfunctionLow) -> [ErrBatterySOCMallfunctionLow]
  BatterySafety/2(ErrBatterySOCMallfunctionHigh) -> [ErrBatterySOCMallfunctionHigh]
  BatterySafety/3(ErrBatteryVoltageLow) -> [ErrBatteryVoltageLow]
  BatterySafety/4(ErrBatteryVoltageHigh) -> [ErrBatteryVoltageHigh]
  BatterySafety/5(ErrBatteryCurrentLow) -> [ErrBatteryCurrentLow]
  BatterySafety/6(ErrBatteryPowerLow) -> [ErrBatteryPowerLow]
  BatterySafety/7(ErrBatteryPowerHigh) -> [ErrBatteryPowerHigh]
  Subsystem/2(ErrVaPSMSVoltageHigh) -> [ErrVaPSMSVoltageHigh]
  Subsystem/3(ErrVbPSMSVoltageLow) -> [ErrVbPSMSVoltageLow]
  Subsystem/4(ErrVbPSMSVoltageHigh) -> [ErrVbPSMSVoltageHigh]
  Subsystem/5(ErrVcPSMSVoltageLow) -> [ErrVcPSMSVoltageLow]
  Subsystem/6(ErrVcPSMSVoltageHigh) -> [ErrVcPSMSVoltageHigh]
  Subsystem/7(ErrAplhaVoltageLow) -> [ErrAplhaVoltageLow]
  Subsystem/8(ErrAlphaVoltageHigh) -> [ErrAlphaVoltageHigh]
  Subsystem/10(ErrBetaVoltageHigh) -> [ErrBetaVoltageHigh]
  Subsystem/9(ErrBetaVoltageLow) -> [ErrBetaVoltageLow]
  [Ds] -> Subsystem2/1(Ds)
  [Qs] -> Subsystem2/2(Qs)
  [InvAlpha] -> Subsystem2/3(InvAlpha)
  [InvBeta] -> Subsystem2/4(InvBeta)
  [VaPulse] -> Subsystem2/5(VaPulse)
  [VbPulse] -> Subsystem2/6(VbPulse)
  [VcPulse] -> Subsystem2/7(VcPulse)
  [cosIn] -> Subsystem2/8(cosIn)
  [sinIn] -> Subsystem2/9(sinIn)
  Subsystem1/1(ErrSpeedVoltageLow) -> [ErrSpeedVoltageLow]
  Subsystem1/5(ErrIqLow) -> [ErrIqLow]
  Subsystem1/6(ErrIqHigh) -> [ErrIqHigh]
  Subsystem1/4(ErrIdHigh) -> [ErrIdHigh]
  Subsystem1/2(ErrSpeedVoltageHigh) -> [ErrSpeedVoltageHigh]
  Subsystem1/3(ErrIdLow) -> [ErrIdLow]
  Subsystem2/1(ErrDsLow) -> [ErrDsLow]
  Subsystem2/2(ErrDsHigh) -> [ErrDsHigh]
  Subsystem2/3(ErrQsLow) -> [ErrQsLow]
  Subsystem2/4(ErrQsHigh) -> [ErrQsHigh]
  Subsystem2/5(ErrAlphaInvLow) -> [ErrAlphaInvLow]
  Subsystem2/6(ErrAlphaInvHigh) -> [ErrAlphaInvHigh]
  Subsystem2/7(ErrBetaInvLow) -> [ErrBetaInvLow]
  Subsystem2/8(ErrBetaInvHigh) -> [ErrBetaInvHigh]
  Subsystem2/9(ErrVaPulseLow) -> [ErrVaPulseLow]
  Subsystem2/10(ErrVaPulseHigh) -> [ErrVaPulseHigh]
  Subsystem2/11(ErrVbPulseLow) -> [ErrVbPulseLow]
  Subsystem2/12(ErrVbPulseHigh) -> [ErrVbPulseHigh]
  Subsystem2/13(ErrVcPulseLow) -> [ErrVcPulseLow]
  Subsystem2/14(ErrVcPulseHigh) -> [ErrVcPulseHigh]
  Subsystem2/15(ErrCosineLow) -> [ErrCosineLow]
  Subsystem2/16(ErrCosineHigh) -> [ErrCosineHigh]
  Subsystem2/17(ErrSineLow) -> [ErrSineLow]
  Subsystem2/18(ErrSineHigh) -> [ErrSineHigh]
  [ErrTriFazicLow] -> Bus Creator/1
  [ErrTriFazicHigh] -> Bus Creator/2
  [ErrTriFazicOverCurrent] -> Bus Creator/3
  [ErrTriFazicLowVoltage] -> Bus Creator/4
  [ErrTriFazicHighVoltage] -> Bus Creator/5
  [ErrDCDCBoostOverVoltage] -> Bus Creator/6
  [ErrDCDCBoostInputVoltageLow] -> Bus Creator/7
  [ErrDCDCBoostInputVoltageHigh] -> Bus Creator/8
  [ErrBatterySOCMallfunctionLow] -> Bus Creator/9
  [ErrBatterySOCMallfunctionHigh] -> Bus Creator/10
  [ErrBatteryVoltageLow] -> Bus Creator/11
  [ErrBatteryVoltageHigh] -> Bus Creator/12
  [ErrBatteryCurrentLow] -> Bus Creator/13
  [ErrBatteryPowerLow] -> Bus Creator/14
  [ErrBatteryPowerHigh] -> Bus Creator/15
  [ErrVaPSMSVoltageLow] -> Bus Creator/16
  [ErrVaPSMSVoltageHigh] -> Bus Creator/17
  [ErrVbPSMSVoltageLow] -> Bus Creator/18
  [ErrVbPSMSVoltageHigh] -> Bus Creator/19
  [ErrVcPSMSVoltageLow] -> Bus Creator/20
  [ErrVcPSMSVoltageHigh] -> Bus Creator/21
  [ErrAplhaVoltageLow] -> Bus Creator/22
  [ErrAlphaVoltageHigh] -> Bus Creator/23
  [ErrBetaVoltageLow] -> Bus Creator/24
  [ErrBetaVoltageHigh] -> Bus Creator/25
  [ErrSpeedVoltageLow] -> Bus Creator/26
  [ErrSpeedVoltageHigh] -> Bus Creator/27
  [ErrIdLow] -> Bus Creator/28
  [ErrIdHigh] -> Bus Creator/29
  [ErrIqLow] -> Bus Creator/30
  [ErrIqHigh] -> Bus Creator/31
  [ErrDsLow] -> Bus Creator/32
  [ErrDsHigh] -> Bus Creator/33
  [ErrQsLow] -> Bus Creator/34
  [ErrQsHigh] -> Bus Creator/35
  [ErrAlphaInvLow] -> Bus Creator/36
  [ErrAlphaInvHigh] -> Bus Creator/37
  [ErrBetaInvLow] -> Bus Creator/38
  [ErrBetaInvHigh] -> Bus Creator/39
  [ErrVaPulseLow] -> Bus Creator/40
  [ErrVaPulseHigh] -> Bus Creator/41
  [ErrVbPulseLow] -> Bus Creator/42
  [ErrVbPulseHigh] -> Bus Creator/43
  [ErrVcPulseLow] -> Bus Creator/44
  [ErrVcPulseHigh] -> Bus Creator/45
  [ErrCosineLow] -> Bus Creator/46
  [ErrCosineHigh] -> Bus Creator/47
  [ErrSineLow] -> Bus Creator/48
  [ErrSineHigh] -> Bus Creator/49
  RectifierSafety/2(ErrTriFazicHigh) -> [ErrTriFazicHigh]
  Subsystem/1(ErrVaPSMSVoltageLow) -> [ErrVaPSMSVoltageLow]

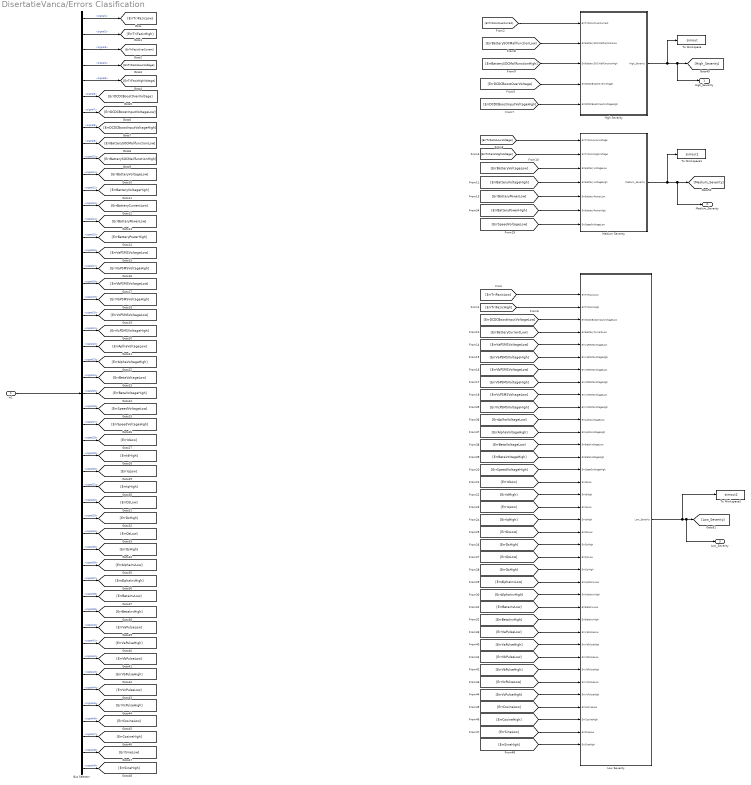
== system DisertatieVanca/Errors Clasification ==
  In1 : Inport
  Bus Selector : BusSelector  OutputSignals=signal1,signal2,signal3,signal4,signal5,signal6,signal7,signal8,signal9,signal10,signal11,signal12,signal13,signal14,signal15,signal16,signal17,signal18,signal19,signal20,signal21,signal22,signal23,signal24,signal25,signal26,signal27,signal28,signal29,signal30,signal31,signal32,signal33,signal34,signal35,signal36,signal37,signal38,signal39,signal40,signal41,signal42,signal43,signal44,signal45,signal46,signal47,signal48,signal49
  High Severity : Subsystem
  Low Severity : Subsystem
  Medium Severity : Subsystem
  To Workspace : ToWorkspace  VariableName=simout  SaveFormat=Timeseries  SampleTime=-1
  To Workspace1 : ToWorkspace  VariableName=simout1  SaveFormat=Timeseries  SampleTime=-1
  To Workspace2 : ToWorkspace  VariableName=simout2  SaveFormat=Timeseries  SampleTime=-1
  High_Severity : Outport
  Medium_Severity : Outport  Port=2
  Low_Severity : Outport  Port=3
  wires:
  Bus Selector/1 -> [ErrTriFazicLow]  "<signal1>"
  In1/1 -> Bus Selector/1
  Bus Selector/2 -> [ErrTriFazicHigh]  "<signal2>"
  Bus Selector/3 -> [ErrTriFazicOverCurrent]  "<signal3>"
  Bus Selector/4 -> [ErrTriFazicLowVoltage]  "<signal4>"
  Bus Selector/5 -> [ErrTriFazicHighVoltage]  "<signal5>"
  Bus Selector/6 -> [ErrDCDCBoostOverVoltage]  "<signal6>"
  Bus Selector/7 -> [ErrDCDCBoostInputVoltageLow]  "<signal7>"
  Bus Selector/8 -> [ErrDCDCBoostInputVoltageHigh]  "<signal8>"
  Bus Selector/9 -> [ErrBatterySOCMallfunctionLow]  "<signal9>"
  Bus Selector/10 -> [ErrBatterySOCMallfunctionHigh]  "<signal10>"
  Bus Selector/11 -> [ErrBatteryVoltageLow]  "<signal11>"
  Bus Selector/12 -> [ErrBatteryVoltageHigh]  "<signal12>"
  Bus Selector/13 -> [ErrBatteryCurrentLow]  "<signal13>"
  Bus Selector/14 -> [ErrBatteryPowerLow]  "<signal14>"
  Bus Selector/15 -> [ErrBatteryPowerHigh]  "<signal15>"
  Bus Selector/16 -> [ErrVaPSMSVoltageLow]  "<signal16>"
  Bus Selector/17 -> [ErrVaPSMSVoltageHigh]  "<signal17>"
  Bus Selector/18 -> [ErrVbPSMSVoltageLow]  "<signal18>"
  Bus Selector/19 -> [ErrVbPSMSVoltageHigh]  "<signal19>"
  Bus Selector/20 -> [ErrVcPSMSVoltageLow]  "<signal20>"
  Bus Selector/21 -> [ErrVcPSMSVoltageHigh]  "<signal21>"
  Bus Selector/22 -> [ErrAplhaVoltageLow]  "<signal22>"
  Bus Selector/23 -> [ErrAlphaVoltageHigh]  "<signal23>"
  Bus Selector/24 -> [ErrBetaVoltageLow]  "<signal24>"
  Bus Selector/25 -> [ErrBetaVoltageHigh]  "<signal25>"
  Bus Selector/26 -> [ErrSpeedVoltageLow]  "<signal26>"
  Bus Selector/27 -> [ErrSpeedVoltageHigh]  "<signal27>"
  Bus Selector/28 -> [ErrIdLow]  "<signal28>"
  Bus Selector/29 -> [ErrIdHigh]  "<signal29>"
  Bus Selector/30 -> [ErrIqLow]  "<signal30>"
  Bus Selector/31 -> [ErrIqHigh]  "<signal31>"
  Bus Selector/32 -> [ErrDsLow]  "<signal32>"
  Bus Selector/33 -> [ErrDsHigh]  "<signal33>"
  Bus Selector/34 -> [ErrQsLow]  "<signal34>"
  Bus Selector/35 -> [ErrQsHigh]  "<signal35>"
  Bus Selector/36 -> [ErrAlphaInvLow]  "<signal36>"
  Bus Selector/37 -> [ErrAlphaInvHigh]  "<signal37>"
  Bus Selector/38 -> [ErrBetaInvLow]  "<signal38>"
  Bus Selector/39 -> [ErrBetaInvHigh]  "<signal39>"
  Bus Selector/40 -> [ErrVaPulseLow]  "<signal40>"
  Bus Selector/41 -> [ErrVaPulseHigh]  "<signal41>"
  Bus Selector/42 -> [ErrVbPulseLow]  "<signal42>"
  Bus Selector/43 -> [ErrVbPulseHigh]  "<signal43>"
  Bus Selector/44 -> [ErrVcPulseLow]  "<signal44>"
  Bus Selector/45 -> [ErrVcPulseHigh]  "<signal45>"
  Bus Selector/46 -> [ErrCosineLow]  "<signal46>"
  Bus Selector/47 -> [ErrCosineHigh]  "<signal47>"
  Bus Selector/48 -> [ErrSineLow]  "<signal48>"
  Bus Selector/49 -> [ErrSineHigh]  "<signal49>"
  [ErrTriFazicOverCurrent] -> High Severity/1(ErrTriFazicOverCurrent)
  [ErrBatterySOCMallfunctionLow] -> High Severity/2(ErrBatterySOCMallfunctionLow)
  [ErrBatterySOCMallfunctionHigh] -> High Severity/3(ErrBatterySOCMallfunctionHigh)
  [ErrDCDCBoostOverVoltage] -> High Severity/4(ErrDCDCBoostOverVoltage)
  [ErrDCDCBoostInputVoltageHigh] -> High Severity/5(ErrDCDCBoostInputVoltageHigh)
  [ErrTriFazicLowVoltage] -> Medium Severity/1(ErrTriFazicLowVoltage)
  [ErrTriFazicHighVoltage] -> Medium Severity/2(ErrTriFazicHighVoltage)
  [ErrBatteryVoltageLow] -> Medium Severity/3(ErrBatteryVoltageLow)
  [ErrBatteryVoltageHigh] -> Medium Severity/4(ErrBatteryVoltageHigh)
  [ErrBatteryPowerLow] -> Medium Severity/5(ErrBatteryPowerLow)
  [ErrBatteryPowerHigh] -> Medium Severity/6(ErrBatteryPowerHigh)
  [ErrSpeedVoltageLow] -> Medium Severity/7(ErrSpeedVoltageLow)
  [ErrTriFazicLow] -> Low Severity/1(ErrTriFazicLow)
  [ErrTriFazicHigh] -> Low Severity/2(ErrTriFazicHigh)
  [ErrDCDCBoostInputVoltageLow] -> Low Severity/3(ErrDCDCBoostInputVoltageLow)
  [ErrBatteryCurrentLow] -> Low Severity/4(ErrBatteryCurrentLow)
  [ErrVaPSMSVoltageLow] -> Low Severity/5(ErrVaPSMSVoltageLow)
  [ErrVaPSMSVoltageHigh] -> Low Severity/6(ErrVaPSMSVoltageHigh)
  [ErrVbPSMSVoltageLow] -> Low Severity/7(ErrVbPSMSVoltageLow)
  [ErrVbPSMSVoltageHigh] -> Low Severity/8(ErrVbPSMSVoltageHigh)
  [ErrVcPSMSVoltageLow] -> Low Severity/9(ErrVcPSMSVoltageLow)
  [ErrVcPSMSVoltageHigh] -> Low Severity/10(ErrVcPSMSVoltageHigh)
  [ErrAplhaVoltageLow] -> Low Severity/11(ErrAplhaVoltageLow)
  [ErrAlphaVoltageHigh] -> Low Severity/12(ErrAlphaVoltageHigh)
  [ErrBetaVoltageLow] -> Low Severity/13(ErrBetaVoltageLow)
  [ErrBetaVoltageHigh] -> Low Severity/14(ErrBetaVoltageHigh)
  [ErrSpeedVoltageHigh] -> Low Severity/15(ErrSpeedVoltageHigh)
  [ErrIdLow] -> Low Severity/16(ErrIdLow)
  [ErrIdHigh] -> Low Severity/17(ErrIdHigh)
  [ErrIqLow] -> Low Severity/18(ErrIqLow)
  [ErrIqHigh] -> Low Severity/19(ErrIqHigh)
  [ErrDsLow] -> Low Severity/20(ErrDsLow)
  [ErrDsHigh] -> Low Severity/21(ErrDsHigh)
  [ErrQsLow] -> Low Severity/22(ErrQsLow)
  [ErrQsHigh] -> Low Severity/23(ErrQsHigh)
  [ErrAlphaInvLow] -> Low Severity/24(ErrAlphaInvLow)
  [ErrAlphaInvHigh] -> Low Severity/25(ErrAlphaInvHigh)
  [ErrBetaInvLow] -> Low Severity/26(ErrBetaInvLow)
  [ErrBetaInvHigh] -> Low Severity/27(ErrBetaInvHigh)
  [ErrVaPulseLow] -> Low Severity/28(ErrVaPulseLow)
  [ErrVaPulseHigh] -> Low Severity/29(ErrVaPulseHigh)
  [ErrVbPulseLow] -> Low Severity/30(ErrVbPulseLow)
  [ErrVbPulseHigh] -> Low Severity/31(ErrVbPulseHigh)
  [ErrVcPulseLow] -> Low Severity/32(ErrVcPulseLow)
  [ErrVcPulseHigh] -> Low Severity/33(ErrVcPulseHigh)
  [ErrCosineLow] -> Low Severity/34(ErrCosineLow)
  [ErrCosineHigh] -> Low Severity/35(ErrCosineHigh)
  [ErrSineLow] -> Low Severity/36(ErrSineLow)
  [ErrSineHigh] -> Low Severity/37(ErrSineHigh)
  High Severity/1(High_Severity) -> To Workspace/1, High_Severity/1, [High_Severity]
  Medium Severity/1(Medium_Severity) -> To Workspace1/1, Medium_Severity/1, [Medium_Severity]
  Low Severity/1(Low_Severity) -> To Workspace2/1, Low_Severity/1, [Low_Severity]

== system DisertatieVanca/Park trans. ==
  note: DQ transformation
  alpha : Inport
  Beta : Inport  Port=2
  sin : Inport  Port=3
  cos : Inport  Port=4
  Add : Sum
  Add1 : Sum  Inputs=-+
  Divide{,1..3} (4 alike) : Product  Inputs=**
  D : Outport
  Q : Outport  Port=2
  wires:
  cos/1 -> Divide/1, Divide3/1
  Divide3/1 -> Add1/1
  alpha/1 -> Divide2/2, Divide/2
  Divide1/1 -> Add/1
  sin/1 -> Divide2/1, Divide1/1
  Add1/1 -> Q/1
  Divide/1 -> Add/2
  Divide2/1 -> Add1/2
  Beta/1 -> Divide3/2, Divide1/2
  Add/1 -> D/1

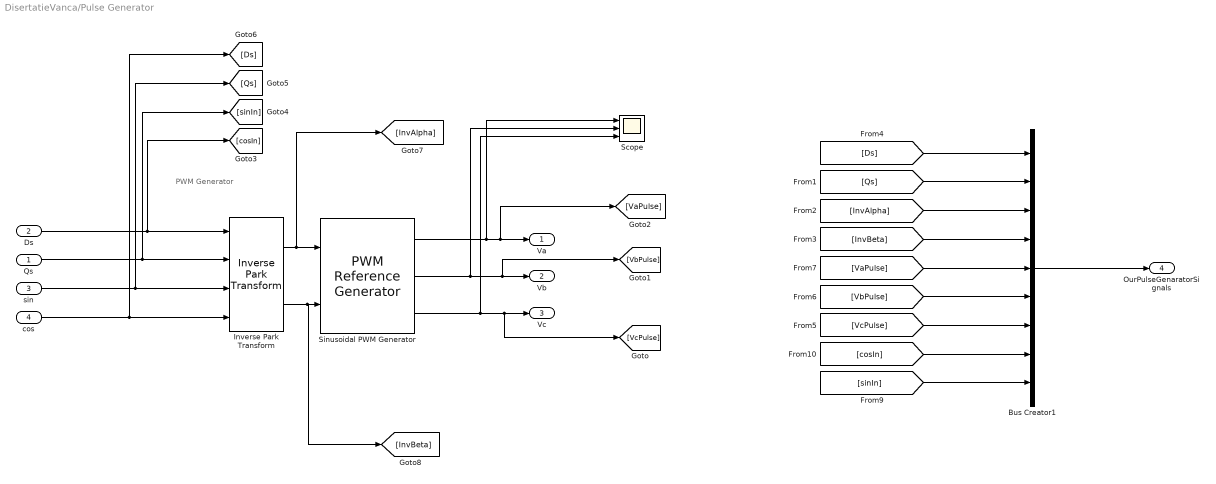
== system DisertatieVanca/Pulse Generator ==
  note: PWM Generator
  Qs : Inport
  Ds : Inport  Port=2
  sin : Inport  Port=3
  cos : Inport  Port=4
  Bus Creator1 : BusCreator  Inputs=9
  Inverse Park Transform : mcbcontrolslib/Inverse Park Transform  AxisAlignment=D-axis
  Scope : Scope  NumInputPorts=3
  Sinusoidal PWM Generator : mcbcontrolslib/PWM Reference Generator  inSignal=Valphabeta  modType=SPWM: sinusoidal PWM
  Va : Outport
  Vb : Outport  Port=2
  Vc : Outport  Port=3
  OurPulseGenaratorSignals : Outport  Port=4
  wires:
  Inverse Park Transform/2 -> Sinusoidal PWM Generator/2, [InvBeta]
  Inverse Park Transform/1 -> [InvAlpha], Sinusoidal PWM Generator/1
  cos/1 -> [Ds], Inverse Park Transform/4
  Qs/1 -> [sinIn], Inverse Park Transform/2
  sin/1 -> [Qs], Inverse Park Transform/3
  Ds/1 -> [cosIn], Inverse Park Transform/1
  Sinusoidal PWM Generator/1 -> Scope/1, [VaPulse], Va/1
  Sinusoidal PWM Generator/2 -> Scope/2, [VbPulse], Vb/1
  Sinusoidal PWM Generator/3 -> Scope/3, [VcPulse], Vc/1
  Bus Creator1/1 -> OurPulseGenaratorSignals/1
  [Ds] -> Bus Creator1/1
  [Qs] -> Bus Creator1/2
  [InvAlpha] -> Bus Creator1/3
  [InvBeta] -> Bus Creator1/4
  [VaPulse] -> Bus Creator1/5
  [VbPulse] -> Bus Creator1/6
  [VcPulse] -> Bus Creator1/7
  [cosIn] -> Bus Creator1/8
  [sinIn] -> Bus Creator1/9

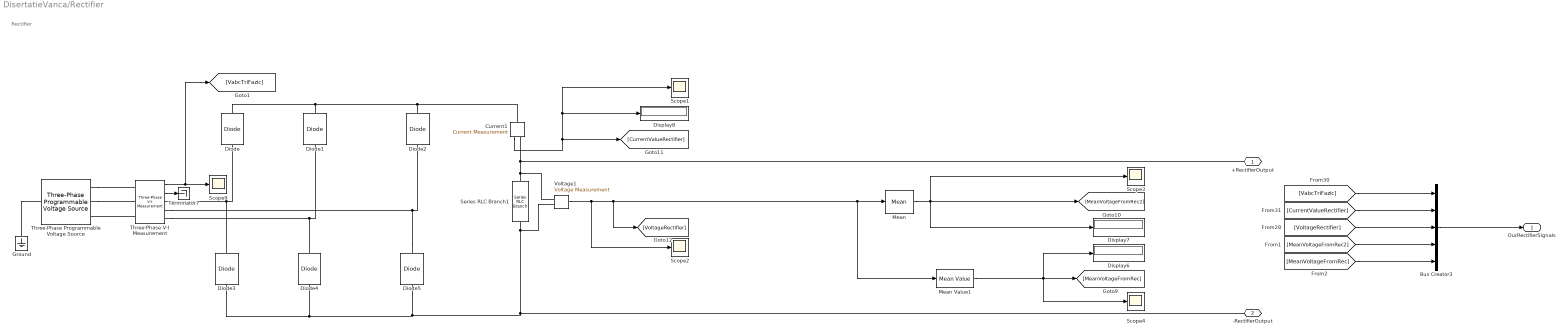
== system DisertatieVanca/Rectifier ==
  note: Rectifier
  Bus Creator3 : BusCreator  Inputs=5
  Current1 : spsCurrentMeasurementLib/Current Measurement  PhasorSimulation=off  OutputType=Complex  PSBequivalent=0
  Diode{,1..5} (6 alike) : spsDiodeLib/Diode  Ron=0.001  Lon=0  Vf=0.8  IC=0  UseSnubber=off  Rs=500  Cs=250e-9  Measurements=off
  Display6 : Display
  Display7 : Display
  Display8 : Display
  Ground : spsGroundLib/Ground  LConnTagsString=a
  Mean : spsMeanLib/Mean  Freq=50  Vinit=0  Ts=0
  Mean Value1 : powerlib_extras/Measurements/Mean Value  Period=1/50
  Scope{1..4,9} (5 alike) : Scope
  Series RLC Branch1 : spsSeriesRLCBranchLib/Series RLC Branch  LConnTagsString=__new0  RConnTagsString=__new0  BranchType=R  Resistance=1  Inductance=80e-3  SetiL0=off  InitialCurrent=0  Capacitance=1e-6  Setx0=off  InitialVoltage=0  Measurements=None
  Terminator7 : Terminator
  Three-Phase Programmable Voltage Source : spsThreePhaseProgrammableVoltageSourceLib/Three-Phase Programmable Voltage Source  PositiveSequence="[400  0 50]"  VariationEntity=None  VariationType=Table of time-amplitude pairs  VariationTypeAlt=Step  VariationStep=0.5  VariationRate=10  VariationMagnitude=0.3  VariationFrequency=2  VariationTiming=[1 2]  VariationPhaseA=off  Amplitudes=[1 0.8 1.2 1.0]  TimeValues=[0 0.1 0.15 0.2]  HarmonicGeneration=off  HarmonicA=[3 0.2 -25 0]  HarmonicB=[2 0.15 35 2]  Timing="[0.05  3]"  BusType=swing  Pref=0  Qref=0  Qmin=-inf  Qmax=inf
  Three-Phase V-I Measurement : spsThreePhaseVIMeasurementLib/Three-Phase V-I Measurement  VoltageMeasurement=phase-to-ground  SetLabelV=off  LabelV=Vabc  Vpu=off  VpuLL=off  CurrentMeasurement=yes  SetLabelI=off  LabelI=Iabc  Ipu=off  Pbase=100e6  Vbase=500e3  OutputType=Complex  PhasorSimulation=off  PSBequivalent=0
  Voltage1 : spsVoltageMeasurementLib/Voltage Measurement  PhasorSimulation=off  OutputType=Complex  PSBequivalent=0
  +RectifierOutput : PMIOPort  Side=Right
  -RectifierOutput : PMIOPort  Port=2  Side=Right
  OurRectifierSignals : Outport
  wires:
  Current1/1 -> Scope1/1, Display8/1, [CurrentValueRectifier]
  Voltage1/1 -> [VoltageRectifier], Mean Value1/1, Mean/1, Scope2/1
  Mean/1 -> [MeanVoltageFromRec2], Display7/1, Scope3/1
  Three-Phase V-I Measurement/2 -> Terminator7/1
  Mean Value1/1 -> [MeanVoltageFromRec], Display6/1, Scope4/1
  Three-Phase V-I Measurement/1 -> [VabcTriFazic], Scope9/1
  [VoltageRectifier] -> Bus Creator3/3
  [VabcTriFazic] -> Bus Creator3/1
  [CurrentValueRectifier] -> Bus Creator3/2
  Bus Creator3/1 -> OurRectifierSignals/1
  [MeanVoltageFromRec2] -> Bus Creator3/4
  [MeanVoltageFromRec] -> Bus Creator3/5
  connections:
  Diode5/RConn1 -- Diode2/LConn1 -- Three-Phase V-I Measurement/RConn2
  Diode3/RConn1 -- Diode/LConn1 -- Three-Phase V-I Measurement/RConn1
  Diode2/RConn1 -- Current1/LConn1 -- Diode/RConn1 -- Diode1/RConn1
  Voltage1/LConn1 -- +RectifierOutput/RConn1 -- Current1/RConn1 -- Series RLC Branch1/LConn1
  Diode4/RConn1 -- Diode1/LConn1 -- Three-Phase V-I Measurement/RConn3
  Ground/LConn1 -- Three-Phase Programmable Voltage Source/LConn1
  Voltage1/LConn2 -- Series RLC Branch1/RConn1 -- Diode5/LConn1 -- Diode3/LConn1 -- Diode4/LConn1 -- -RectifierOutput/RConn1
  Three-Phase V-I Measurement/LConn3 -- Three-Phase Programmable Voltage Source/RConn3
  Three-Phase Programmable Voltage Source/RConn2 -- Three-Phase V-I Measurement/LConn2
  Three-Phase Programmable Voltage Source/RConn1 -- Three-Phase V-I Measurement/LConn1

== system DisertatieVanca/Reinforcement Learning ==
  id : Inport
  iq : Inport  Port=2
  id ref : Inport  Port=3
  iq ref : Inport  Port=4
  speed ref : Inport  Port=5
  speed fb : Inport  Port=6
  Bus Creator1 : BusCreator  Inputs=6
  Data Type Conversion : DataTypeConversion  OutDataTypeStr=dataType  SaturateOnIntegerOverflow=off  RndMeth=Floor
  Data Type Conversion1 : DataTypeConversion  OutDataTypeStr=double  SaturateOnIntegerOverflow=off  RndMeth=Floor
  IsDone : Subsystem
  Observations : Subsystem
  RL Agent : rllib/RL Agent  Agent=agent  ExternalActionAsInput=off  ProvideLastAction=off  ProvideCumRwd=off  TreatAsDirectFeedthrough=on  UseStrictObservationDataTypes=off
  Reward : Subsystem
  Sum : Sum  Inputs=|+-  OutDataTypeStr=Inherit: Inherit via back propagation
  Sum1 : Sum  Inputs=|+-  OutDataTypeStr=Inherit: Inherit via back propagation
  Unit Delay2 : UnitDelay  SampleTime=-1  HasFrameUpgradeWarning=on
  action : Outport
  OutRfSignals : Outport  Port=2
  wires:
  Data Type Conversion1/1 -> Observations/1(speed ref)
  Data Type Conversion/1 -> action/1
  IsDone/1(stop) -> Reward/3(done), RL Agent/3
  RL Agent/1 -> Unit Delay2/1, Data Type Conversion/1
  Unit Delay2/1 -> Reward/4(action)
  id ref/1 -> Sum/1, [IdRef]
  id/1 -> [Id_], Sum/2, Observations/4(id)
  iq ref/1 -> [IqRef], Sum1/1, IsDone/1(Iq_ref)
  Observations/1(observations) -> RL Agent/1
  Reward/1(reward) -> RL Agent/2
  speed ref/1 -> [speed_ref], Data Type Conversion1/1
  speed fb/1 -> [speed_fb], Observations/2(speed fb)
  iq/1 -> [Iq_], Observations/6(iq), Sum1/2
  Sum/1 -> Reward/1(id error), Observations/3(id err)
  Sum1/1 -> Observations/5(iq err), Reward/2(iq error)
  Bus Creator1/1 -> OutRfSignals/1
  [IdRef] -> Bus Creator1/1
  [IqRef] -> Bus Creator1/2
  [Id_] -> Bus Creator1/3
  [Iq_] -> Bus Creator1/4
  [speed_fb] -> Bus Creator1/5
  [speed_ref] -> Bus Creator1/6

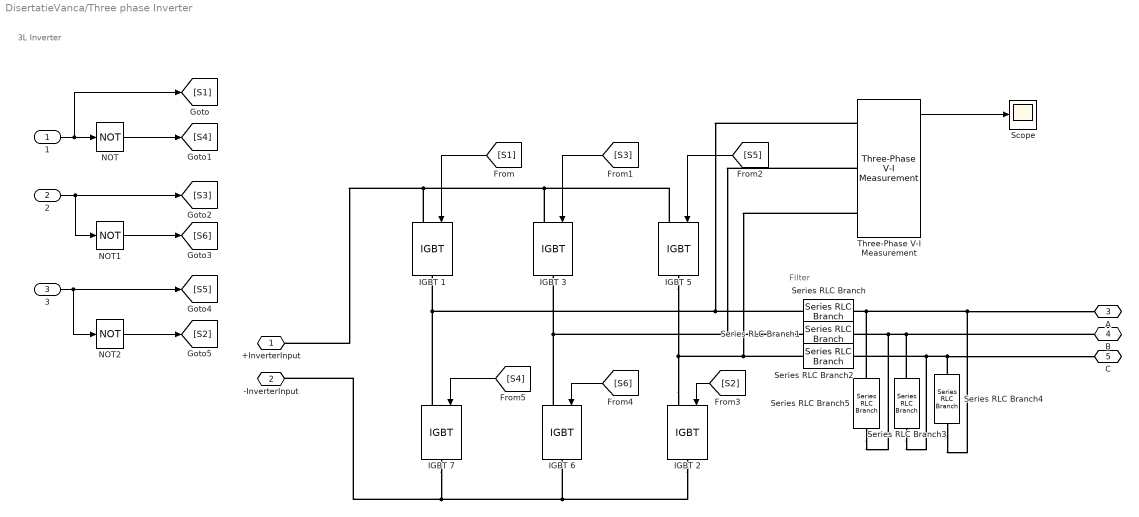
== system DisertatieVanca/Three phase Inverter ==
  note: Filter
  note: 3L Inverter
  1 : Inport
  2 : Inport  Port=2
  3 : Inport  Port=3
  IGBT {1..3,5..7} (6 alike) : spsIGBTLib/IGBT  Ron=0.001  Lon=0  Vf=1  Tf=1e-6  Tt=2e-6  IC=0  Rs=1e5  Cs=inf  Measurements=off
  NOT : Logic  Operator=NOT  IconShape=distinctive  AllPortsSameDT=off  OutDataTypeStr=boolean
  NOT1 : Logic  Operator=NOT  IconShape=distinctive  AllPortsSameDT=off  OutDataTypeStr=boolean
  NOT2 : Logic  Operator=NOT  IconShape=distinctive  AllPortsSameDT=off  OutDataTypeStr=boolean
  Scope : Scope
  Series RLC Branch : spsSeriesRLCBranchLib/Series RLC Branch  LConnTagsString=__new0  RConnTagsString=__new0  BranchType=L  Resistance=1  Inductance=470e-6  SetiL0=off  InitialCurrent=0  Capacitance=1e-6  Setx0=off  InitialVoltage=0  Measurements=None
  Series RLC Branch1 : spsSeriesRLCBranchLib/Series RLC Branch  LConnTagsString=__new0  RConnTagsString=__new0  BranchType=L  Resistance=1  Inductance=470e-6  SetiL0=off  InitialCurrent=0  Capacitance=1e-6  Setx0=off  InitialVoltage=0  Measurements=None
  Series RLC Branch2 : spsSeriesRLCBranchLib/Series RLC Branch  LConnTagsString=__new0  RConnTagsString=__new0  BranchType=L  Resistance=1  Inductance=470e-6  SetiL0=off  InitialCurrent=0  Capacitance=1e-6  Setx0=off  InitialVoltage=0  Measurements=None
  Series RLC Branch3 : spsSeriesRLCBranchLib/Series RLC Branch  LConnTagsString=__new0  RConnTagsString=__new0  BranchType=C  Resistance=1  Inductance=1e-3  SetiL0=off  InitialCurrent=0  Capacitance=1e-6  Setx0=off  InitialVoltage=0  Measurements=None
  Series RLC Branch4 : spsSeriesRLCBranchLib/Series RLC Branch  LConnTagsString=__new0  RConnTagsString=__new0  BranchType=C  Resistance=1  Inductance=1e-3  SetiL0=off  InitialCurrent=0  Capacitance=1e-6  Setx0=off  InitialVoltage=0  Measurements=None
  Series RLC Branch5 : spsSeriesRLCBranchLib/Series RLC Branch  LConnTagsString=__new0  RConnTagsString=__new0  BranchType=C  Resistance=1  Inductance=1e-3  SetiL0=off  InitialCurrent=0  Capacitance=1e-6  Setx0=off  InitialVoltage=0  Measurements=None
  "Three-Phase V-I Measurement " : spsThreePhaseVIMeasurementLib/Three-Phase V-I Measurement  VoltageMeasurement=phase-to-phase  SetLabelV=off  LabelV=Vabc  Vpu=off  VpuLL=off  CurrentMeasurement=no  SetLabelI=off  LabelI=Iabc  Ipu=off  Pbase=100e6  Vbase=500e3  OutputType=Complex  PhasorSimulation=off  PSBequivalent=0
  +InverterInput : PMIOPort  Side=Left
  -InverterInput : PMIOPort  Port=2  Side=Left
  A : PMIOPort  Port=3  Side=Right
  B : PMIOPort  Port=4  Side=Right
  C : PMIOPort  Port=5  Side=Right
  wires:
  [S3] -> IGBT 3/1
  [S1] -> IGBT 1/1
  [S5] -> IGBT 5/1
  [S4] -> IGBT 7/1
  [S6] -> IGBT 6/1
  [S2] -> IGBT 2/1
  1/1 -> [S1], NOT/1
  NOT/1 -> [S4]
  2/1 -> [S3], NOT1/1
  NOT1/1 -> [S6]
  3/1 -> NOT2/1, [S5]
  NOT2/1 -> [S2]
  "Three-Phase V-I Measurement "/1 -> Scope/1
  connections:
  IGBT 3/RConn1 -- "Three-Phase V-I Measurement "/LConn2 -- Series RLC Branch1/LConn1 -- IGBT 6/LConn1
  IGBT 6/RConn1 -- IGBT 2/RConn1 -- IGBT 7/RConn1 -- -InverterInput/RConn1
  Series RLC Branch2/RConn1 -- Series RLC Branch3/RConn1 -- Series RLC Branch4/LConn1 -- C/RConn1
  IGBT 1/RConn1 -- "Three-Phase V-I Measurement "/LConn1 -- Series RLC Branch/LConn1 -- IGBT 7/LConn1
  IGBT 5/LConn1 -- IGBT 3/LConn1 -- IGBT 1/LConn1 -- +InverterInput/RConn1
  IGBT 2/LConn1 -- "Three-Phase V-I Measurement "/LConn3 -- Series RLC Branch2/LConn1 -- IGBT 5/RConn1
  Series RLC Branch4/RConn1 -- A/RConn1 -- Series RLC Branch5/LConn1 -- Series RLC Branch/RConn1
  Series RLC Branch1/RConn1 -- Series RLC Branch5/RConn1 -- B/RConn1 -- Series RLC Branch3/LConn1
